simulink model "BD_CONVAT"  (Simulink 4.1.1)
settings: Solver=ode1  SolverMode=SingleTasking  StartTime=0.0  StopTime=max(cyc_mph(:,1))  FixedStep=1  MaxStep=1  RelTol=1e-3  AbsTol=1e-3
undefined symbols (not defined in the file): ess_on, ex_calc, fc_emis, vc_idle_spd
libraries: lib_transmission x3, lib_wheel x2, lib_help x2, lib_outputs x1, lib_controls x1, lib_interactive x1, lib_accessory x1, lib_drive_cycle x1, lib_exhaust x1, lib_fuel_converter x1, lib_vehicle x1
settings Model: LastModifiedBy=ssprik  ModifiedComment=ssprik -- Wed Sep 24 14:47:00 2003 -- Version 1.24  SaveTime=off  SaveOutput=off  LimitDataPoints=off  UnconnectedLineMsg=none  RTWTemplateMakefile=grt_vc.tmf  ExtModeTrigMode=oneshot  ExtModeArmWhenConnect=off
settings Model: ModifiedHistory=|
  | ssprik -- Wed Sep 24 14:47:00 2003 -- Version 1.24
  | 
  | 
  | mokeefe -- Wed Feb 19 08:44:57 2003 -- Version 1.23
  | 
  | 
  | mokeefe -- Fri Aug 30 07:39:54 2002 -- Version 1.22
  | Changed the input to "mechanical accessory loads <acc>/Mechanical Accessory Loads V2 <acc>" masked parameter input blocks. In R13, the function "not" no longer returns double 1 or double 0 for true and false but instead returns type logical (boolean). Thus, I am now multiplying by double 1 which causes a type conversion to double yielding the desired effect.
  | 
  | 
  | abrooker -- Tue May 14 11:42:41 2002 -- Version 1.21
  | 
  | 
  | mokeefe -- Thu Apr 18 07:38:59 2002 -- Version 1.20
  | saving the model:
  | o "without the model browser open"
  | o with only top-level screen visible
  | o and with "fit to view" enabled
  | 
  | mokeefe -- Fri Mar 29 15:47:48 2002 -- Version 1.19
  | 
  | 
  | mokeefe -- Wed Mar 06 11:57:40 2002 -- Version 1.18
  | 
  | 
  | mokeefe -- Tue Mar 05 14:28:45 2002 -- Version 1.17
  | 
  | 
  | mokeefe -- Mon Mar 04 15:00:28 2002 -- Version 1.16
  | 
  | 
  | mokeefe -- Fri Mar 01 10:28:47 2002 -- Version 1.15
  | 
  | 
  | mokeefe -- Thu Feb 28 09:24:37 2002 -- Version 1.14
  | 
  | 
  | mokeefe -- Thu Feb 28 09:24:09 2002 -- Version 1.13
  | added in new mask for Mechanical Accessory Loads <acc> (cosmetic change)
  | 
  | mokeefe -- Tue Feb 19 09:32:54 2002 -- Version 1.12
  | 
  | 
  | Adding the Mechanical Accessory driveline block

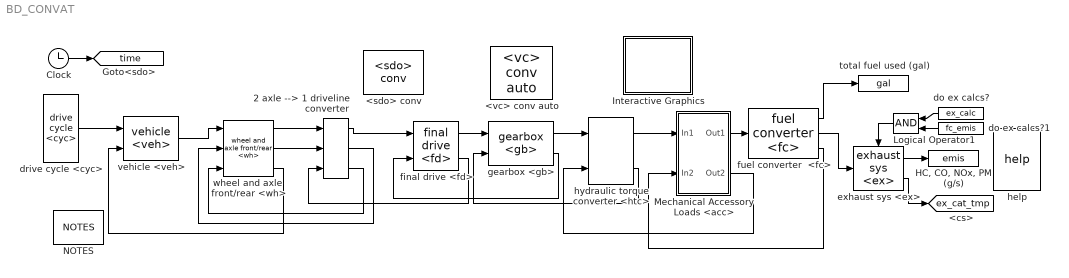
== system BD_CONVAT ==
  2 axle --> 1 driveline converter : lib_wheel/2 axle --> 1 driveline converter
      settings: RTWFcnNameOpts=Auto  RTWFileNameOpts=Auto
  <sdo> conv : lib_outputs/<sdo> conv
  <vc> conv auto : lib_controls/<vc> conv auto
  Clock : Clock
      settings: DisplayTime=off  Decimation=10
  "HC, CO, NOx, PM (g/s)" : ToWorkspace  VariableName=emis  SampleTime=0  SaveFormat=Array
  Interactive Graphics : Subsystem  BlockChoice=off
      settings: AttributesFormatString=%<BlockChoice>  TemplateBlock=lib_interactive/Interactive Graphics  MemberBlocks=off,on  RTWFcnNameOpts=Auto  RTWFileNameOpts=Auto
  Logical Operator1 : Logic  Orientation=left  Operator=AND  Inputs=2
  Mechanical Accessory Loads <acc> : Subsystem
      settings: RTWFcnNameOpts=Auto  RTWFileNameOpts=Auto
      mask Display: image(imread('bdi_acc_pic.bmp'))
  NOTES : lib_help/NOTES
  do ex calcs? : Constant  Orientation=left  Value=ex_calc
  do ex calcs?1 : Constant  Orientation=left  Value=fc_emis
  drive cycle <cyc> : lib_drive_cycle/drive cycle <cyc>
  exhaust sys <ex> : lib_exhaust/exhaust sys <ex>
  final drive <fd> : lib_transmission/final drive <fd>
  fuel converter  <fc> : lib_fuel_converter/fuel converter  <fc>
      link override fuel use and EO emis Configurable Subsystem: BlockChoice=fuel use and EO emis
  gearbox <gb> : lib_transmission/gearbox <gb>
  help : lib_help/help
  hydraulic torque converter <htc> : lib_transmission/hydraulic torque converter <htc>
  total fuel used (gal) : ToWorkspace  VariableName=gal  SampleTime=0  SaveFormat=Array
  vehicle <veh> : lib_vehicle/vehicle <veh>
      link override record achieved force outputs/rolling resistance force: BlockChoice=force req'd to overcome rolling resistance (N) j2452
      link override rolling resistance force: BlockChoice=force req'd to overcome rolling resistance (N) j2452
      link override vehicle speed: BlockChoice=vehicle speed (m/s) j2452
  wheel and axle  front/rear <wh> : lib_wheel/wheel and axle  front//rear <wh>
  tag scope: ex_cat_tmp=global, time=global
  wires:
  wheel and axle  front/rear <wh>/3 -> vehicle <veh>/2
  final drive <fd>/2 -> 2 axle --> 1 driveline converter/3
  final drive <fd>/1 -> gearbox <gb>/1
  gearbox <gb>/2 -> final drive <fd>/2
  Clock/1 -> [time]
  drive cycle <cyc>/1 -> vehicle <veh>/1
  vehicle <veh>/1 -> wheel and axle  front/rear <wh>/1
  gearbox <gb>/1 -> hydraulic torque converter <htc>/1
  hydraulic torque converter <htc>/2 -> gearbox <gb>/2
  fuel converter  <fc>/2 -> exhaust sys <ex>/1
  fuel converter  <fc>/1 -> total fuel used (gal)/1
  exhaust sys <ex>/1 -> "HC, CO, NOx, PM (g/s)"/1
  do ex calcs?/1 -> Logical Operator1/1
  do ex calcs?1/1 -> Logical Operator1/2
  Logical Operator1/1 -> exhaust sys <ex>/Enable
  exhaust sys <ex>/2 -> [ex_cat_tmp]
  hydraulic torque converter <htc>/1 -> Mechanical Accessory Loads <acc>/1(In1)
  Mechanical Accessory Loads <acc>/1(Out1) -> fuel converter  <fc>/1
  Mechanical Accessory Loads <acc>/2(Out2) -> hydraulic torque converter <htc>/2
  fuel converter  <fc>/3 -> Mechanical Accessory Loads <acc>/2(In2)
  wheel and axle  front/rear <wh>/1 -> 2 axle --> 1 driveline converter/1
  wheel and axle  front/rear <wh>/2 -> 2 axle --> 1 driveline converter/2
  2 axle --> 1 driveline converter/1 -> final drive <fd>/1
  2 axle --> 1 driveline converter/3 -> wheel and axle  front/rear <wh>/3
  2 axle --> 1 driveline converter/2 -> wheel and axle  front/rear <wh>/2

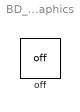
== system BD_CONVAT/Interactive Graphics ==
  off : lib_interactive/off  Tag=Altia_off  Orientation=up

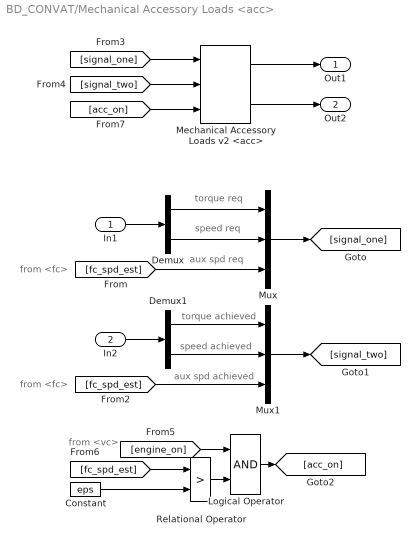
== system BD_CONVAT/Mechanical Accessory Loads <acc> ==
  note: from <fc>
  note: from <fc>
  note: torque req
  note: speed req
  note: aux spd req
  note: torque achieved
  note: speed achieved
  note: aux spd achieved
  note: from <vc>
  In1 : Inport  Port=1  LatchInput=off
  In2 : Inport  Port=2  LatchInput=off
  Constant : Constant  Value=eps
  Demux : Demux  Outputs=2  BusSelectionMode=off
  Demux1 : Demux  Outputs=2  BusSelectionMode=off
  Logical Operator : Logic  Operator=AND  Inputs=2
  Mechanical Accessory Loads v2 <acc> : lib_accessory/Mechanical Accessory Loads v2 <acc>  load_on=not(ess_on)*1  acc_max_spd=inf  acc_min_spd=vc_idle_spd+eps  ic_mech_trq=0  ic_mech_pwr=0
      link override backward model/mechanical accessories (Nm): BlockChoice=Mechanical Accessories: Const Mech Var Elect
      link override estimated mechanical torque/mechanical accessories (Nm): BlockChoice=Mechanical Accessories: Const Mech Var Elect
  Mux : Mux  Inputs=3
  Mux1 : Mux  Inputs=3
  Relational Operator : RelationalOperator  Operator=>
  Out1 : Outport  Port=1
  Out2 : Outport  Port=2
  wires:
  [signal_one] -> Mechanical Accessory Loads v2 <acc>/1
  Mechanical Accessory Loads v2 <acc>/1 -> Out1/1
  Mechanical Accessory Loads v2 <acc>/2 -> Out2/1
  [signal_two] -> Mechanical Accessory Loads v2 <acc>/2
  [acc_on] -> Mechanical Accessory Loads v2 <acc>/3
  Mux/1 -> [signal_one]
  In1/1 -> Demux/1
  Demux/1 -> Mux/1
  Demux/2 -> Mux/2
  [fc_spd_est] -> Mux/3
  Mux1/1 -> [signal_two]
  In2/1 -> Demux1/1
  Demux1/1 -> Mux1/1
  Demux1/2 -> Mux1/2
  [fc_spd_est] -> Mux1/3
  [fc_spd_est] -> Relational Operator/1
  Constant/1 -> Relational Operator/2
  [engine_on] -> Logical Operator/1
  Relational Operator/1 -> Logical Operator/2
  Logical Operator/1 -> [acc_on]
